simulink model "leveller"  (R2025b)
settings: Solver=FixedStepDiscrete  StartTime=0.0  StopTime=inf  FixedStep=128/48000  RelTol=1e-3
model workspace (MATLAB code in the model file):
  | Gain_rt = Simulink.Parameter(1.0);
  | Bypass_rt = Simulink.Parameter(false);
settings Model: Creator=linogarciamorales  LastModifiedBy=linogarciamorales
settings OptimizationCC: EnhancedBackFolding=on  PassReuseOutputArgsAs=Individual arguments  ZeroExternalMemoryAtStartup=off  ZeroInternalMemoryAtStartup=off  OptimizeBlockOrder=speed  DifferentSizesBufferReuse=on  OptimizationCustomize=off  EfficientTunableParamExpr=on
settings DebuggingCC: ParameterTunabilityLossMsg=error
settings SFSimCC: MATLABDynamicMemAlloc=off
settings RTWCC: SystemTargetFile=ert.tlc  GenCodeOnly=on  TemplateMakefile=ert_default_tmf  Description=Embedded Coder
settings CodeAppCC: ForceParamTrailComments=on  IgnoreCustomStorageClasses=off  OperatorAnnotations=on  SimulinkDataObjDesc=on  SFDataObjDesc=on  InsertBlockDesc=on
settings ERTTargetCC: InlinedParameterPlacement=Hierarchical  ERTCustomFileTemplate=example_file_process.tlc  TargetLangStandard=C99 (ISO)  GenerateSampleERTMain=on  SupportNonInlinedSFcns=on

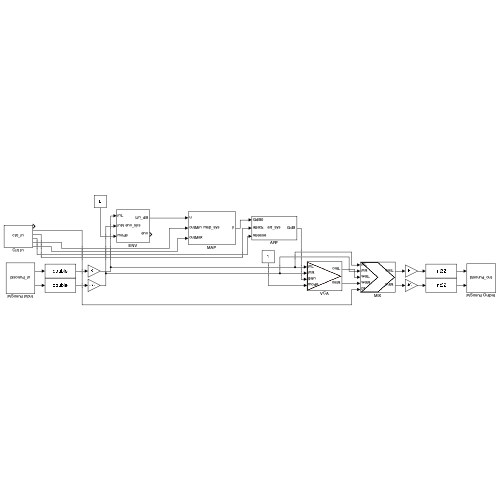
[thumbnail: Simulink's stored preview of the top-level diagram]
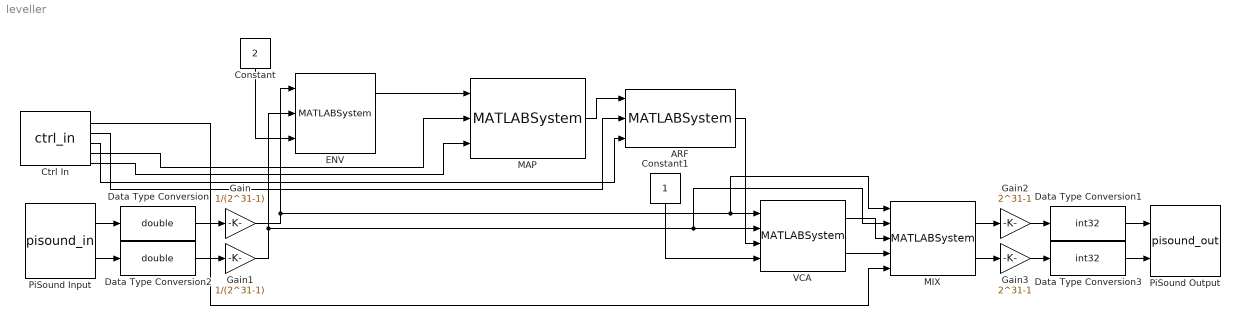
== system leveller ==
  ARF : MATLABSystem  System=arf_sys  N=128  Fs=48000  bypass=uint8(0)  SimulateUsing=Code generation
      mask Type: arf_sys
  Constant : Constant  Value=2  OutDataTypeStr=uint8
  Constant1 : Constant  OutDataTypeStr=uint8
  Ctrl In : S-Function  FunctionName=ctrl_in  Parameters=48000, 128, 6  SFunctionDeploymentMode=off  EnableBusSupport=off
  Data Type Conversion : DataTypeConversion  OutDataTypeStr=double  SaturateOnIntegerOverflow=off  RndMeth=Floor
  Data Type Conversion1 : DataTypeConversion  OutDataTypeStr=int32  SaturateOnIntegerOverflow=off  RndMeth=Floor
  Data Type Conversion2 : DataTypeConversion  OutDataTypeStr=double  SaturateOnIntegerOverflow=off  RndMeth=Floor
  Data Type Conversion3 : DataTypeConversion  OutDataTypeStr=int32  SaturateOnIntegerOverflow=off  RndMeth=Floor
  ENV : MATLABSystem  System=env_sys  N=128  Fs=48000  ModeDefault=uint8( 1 )  Eps=1e-12  TauRMS=0.02  SimulateUsing=Code generation
      mask Type: env_sys
  Gain : Gain  Gain=1/(2^31-1)
  Gain1 : Gain  Gain=1/(2^31-1)
  Gain2 : Gain  Gain=2^31-1
  Gain3 : Gain  Gain=2^31-1
  MAP : MATLABSystem  System=map_sys  bypass=uint8(0)  Mode=uint8(3)  Threshold=-45  Slope=1  SimulateUsing=Code generation  Offset=40
      mask Type: map_sys
  MIX : MATLABSystem  System=mix_sys  N=128  Fs=48000  Mode=uint8( 0 )  SmoothTime=0.01  IndepInDB=false  SimulateUsing=Code generation
      mask Type: mix_sys
  PiSound Input : S-Function  FunctionName=pisound_in  Parameters=48000, 128, 0  SFunctionDeploymentMode=off  EnableBusSupport=off
  PiSound Output : S-Function  FunctionName=pisound_out  Parameters=48000, 128, 0  SFunctionDeploymentMode=off  EnableBusSupport=off
  VCA : MATLABSystem  System=vca_sys  N=128  Fs=48000  bypass=uint8(0)  SimulateUsing=Code generation
      mask Type: vca_sys
  wires:
  PiSound Input/1 -> Data Type Conversion/1
  PiSound Input/2 -> Data Type Conversion2/1
  Data Type Conversion1/1 -> PiSound Output/1
  Data Type Conversion3/1 -> PiSound Output/2
  Gain2/1 -> Data Type Conversion1/1
  Gain3/1 -> Data Type Conversion3/1
  Data Type Conversion/1 -> Gain/1
  Data Type Conversion2/1 -> Gain1/1
  Gain/1 -> ENV/1, MIX/1, VCA/1
  Gain1/1 -> MIX/2, VCA/2, ENV/2
  Constant/1 -> ENV/3
  ENV/1 -> MAP/1
  ARF/1 -> VCA/3
  Constant1/1 -> VCA/4
  MAP/1 -> ARF/1
  VCA/1 -> MIX/3
  VCA/2 -> MIX/4
  MIX/1 -> Gain2/1
  MIX/2 -> Gain3/1
  Ctrl In/2 -> MIX/5
  Ctrl In/3 -> ARF/2
  Ctrl In/4 -> ARF/3
  Ctrl In/5 -> MAP/2
  Ctrl In/6 -> MAP/3
